simulink model "mult_cmpl"  (R2023a)
settings: Solver=VariableStepAuto  StartTime=0.0  StopTime=5  RelTol=1e-3
settings Model: Creator=usradmin  LastModifiedBy=usradmin

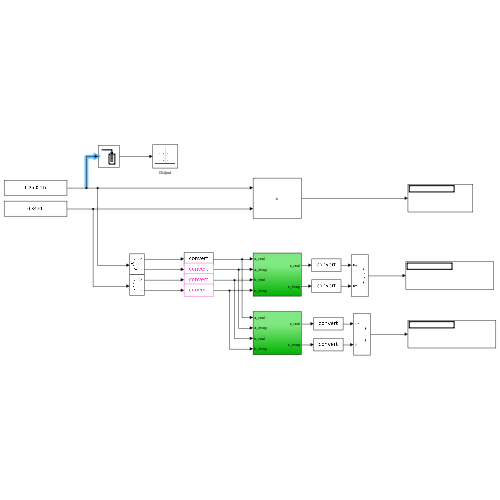
[thumbnail: Simulink's stored preview of the top-level diagram]
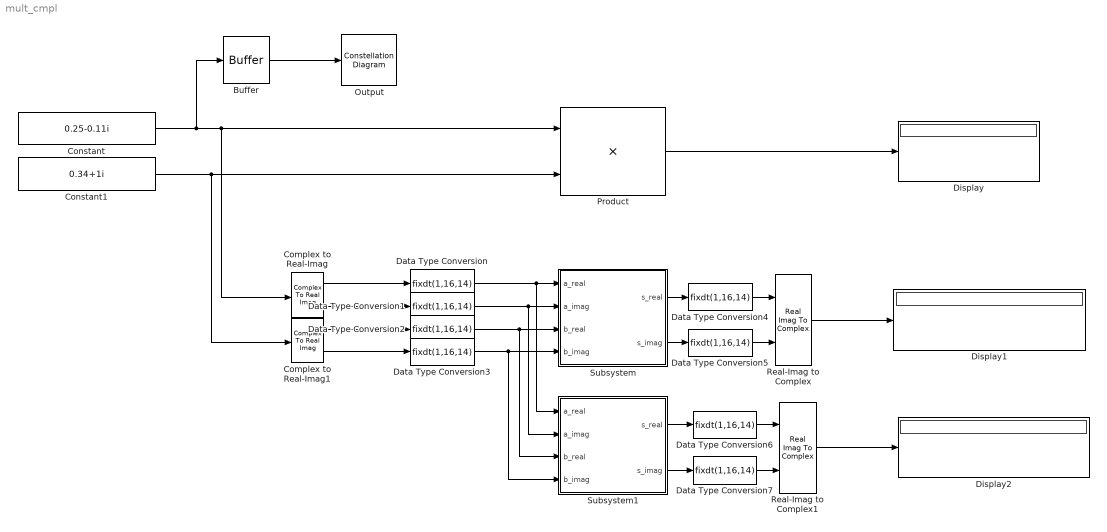
== system mult_cmpl ==
  Buffer : Buffer  N=947*5  OutputFrames=off
  Complex to Real-Imag : ComplexToRealImag
  Complex to Real-Imag1 : ComplexToRealImag
  Constant : Constant  Value=0.25-0.11i
  Constant1 : Constant  Value=0.34+1i
  Data Type Conversion{,1..7} (8 alike) : DataTypeConversion  OutDataTypeStr=fixdt(1,16,14)  SaturateOnIntegerOverflow=off  RndMeth=Floor
  Display : Display
  Display1 : Display
  Display2 : Display
  Output : ConstellationDiagram  WindowPosition=[1891.000000,318.000000,600.000000,600.000000,]  ScopeFrameLocation=window
  Product : Product
  Real-Imag to Complex : RealImagToComplex
  Real-Imag to Complex1 : RealImagToComplex
  Subsystem : Subsystem
  Subsystem1 : Subsystem
  wires:
  Product/1 -> Display/1
  Real-Imag to Complex/1 -> Display1/1
  Constant1/1 -> Complex to Real-Imag1/1, Product/2
  Complex to Real-Imag/1 -> Data Type Conversion/1
  Complex to Real-Imag/2 -> Data Type Conversion1/1
  Complex to Real-Imag1/1 -> Data Type Conversion2/1
  Complex to Real-Imag1/2 -> Data Type Conversion3/1
  Subsystem/1(s_real) -> Data Type Conversion4/1
  Subsystem/2(s_imag) -> Data Type Conversion5/1
  Data Type Conversion/1 -> Subsystem1/1(a_real), Subsystem/1(a_real)
  Data Type Conversion1/1 -> Subsystem1/2(a_imag), Subsystem/2(a_imag)
  Data Type Conversion2/1 -> Subsystem1/3(b_real), Subsystem/3(b_real)
  Data Type Conversion3/1 -> Subsystem1/4(b_imag), Subsystem/4(b_imag)
  Data Type Conversion4/1 -> Real-Imag to Complex/1
  Data Type Conversion5/1 -> Real-Imag to Complex/2
  Data Type Conversion7/1 -> Real-Imag to Complex1/2
  Data Type Conversion6/1 -> Real-Imag to Complex1/1
  Real-Imag to Complex1/1 -> Display2/1
  Subsystem1/1(s_real) -> Data Type Conversion6/1
  Subsystem1/2(s_imag) -> Data Type Conversion7/1
  Buffer/1 -> Output/1
  Constant/1 -> Buffer/1, Complex to Real-Imag/1, Product/1

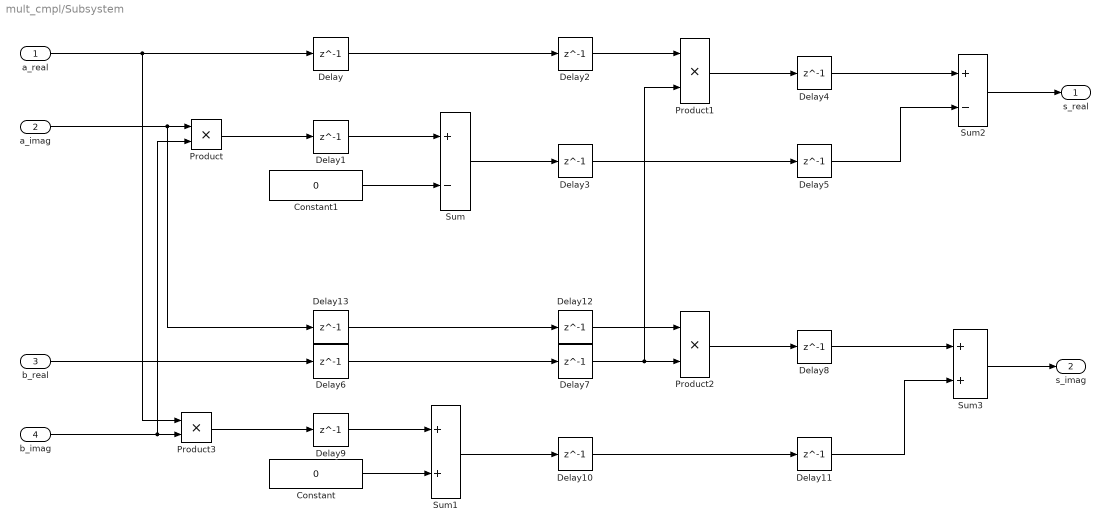
== system mult_cmpl/Subsystem ==
  a_real : Inport
  a_imag : Inport  Port=2
  b_real : Inport  Port=3
  b_imag : Inport  Port=4
  Constant : Constant  Value=0  OutDataTypeStr=fixdt(1,12,11)
  Constant1 : Constant  Value=0  OutDataTypeStr=fixdt(1,12,11)
  Delay{,1..13} (14 alike) : Delay  DelayLength=1  InitialCondition=0
  Product{,1..3} (4 alike) : Product
  Sum : Sum  Inputs=+-
  Sum1 : Sum
  Sum2 : Sum  Inputs=+-
  Sum3 : Sum
  s_real : Outport
  s_imag : Outport  Port=2
  wires:
  a_real/1 -> Delay/1, Product3/1
  a_imag/1 -> Delay13/1, Product/1
  b_imag/1 -> Product3/2, Product/2
  Product/1 -> Delay1/1
  Delay1/1 -> Sum/1
  Delay/1 -> Delay2/1
  Sum/1 -> Delay3/1
  Delay2/1 -> Product1/1
  Product1/1 -> Delay4/1
  Delay4/1 -> Sum2/1
  Delay3/1 -> Delay5/1
  Delay5/1 -> Sum2/2
  Sum2/1 -> s_real/1
  b_real/1 -> Delay6/1
  Delay6/1 -> Delay7/1
  Delay7/1 -> Product1/2, Product2/2
  Product2/1 -> Delay8/1
  Delay8/1 -> Sum3/1
  Sum3/1 -> s_imag/1
  Product3/1 -> Delay9/1
  Delay9/1 -> Sum1/1
  Sum1/1 -> Delay10/1
  Delay10/1 -> Delay11/1
  Delay11/1 -> Sum3/2
  Delay12/1 -> Product2/1
  Delay13/1 -> Delay12/1
  Constant/1 -> Sum1/2
  Constant1/1 -> Sum/2

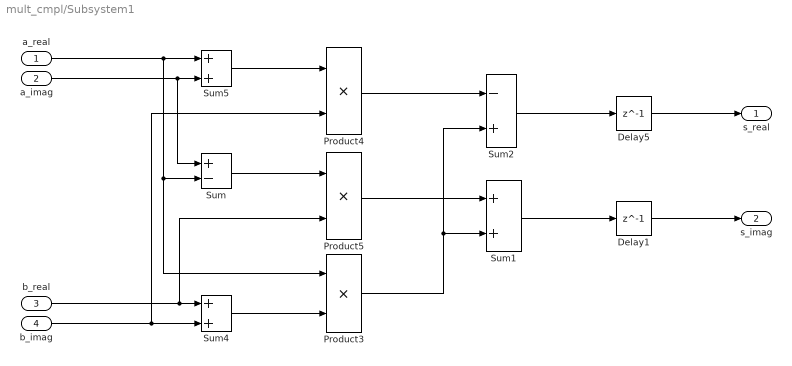
== system mult_cmpl/Subsystem1 ==
  a_real : Inport
  a_imag : Inport  Port=2
  b_real : Inport  Port=3
  b_imag : Inport  Port=4
  Delay1 : Delay  DelayLength=1  InitialCondition=0
  Delay5 : Delay  DelayLength=1  InitialCondition=0
  Product3 : Product
  Product4 : Product
  Product5 : Product
  Sum : Sum  Inputs=+-
  Sum1 : Sum
  Sum2 : Sum  Inputs=-+
  Sum4 : Sum
  Sum5 : Sum
  s_real : Outport
  s_imag : Outport  Port=2
  wires:
  Product3/1 -> Sum1/2, Sum2/2
  Sum1/1 -> Delay1/1
  b_real/1 -> Sum4/1, Product5/2
  Sum2/1 -> Delay5/1
  a_real/1 -> Sum5/1, Product3/1, Sum/2
  b_imag/1 -> Sum4/2, Product4/2
  a_imag/1 -> Sum/1, Sum5/2
  Sum4/1 -> Product3/2
  Sum5/1 -> Product4/1
  Sum/1 -> Product5/1
  Product4/1 -> Sum2/1
  Product5/1 -> Sum1/1
  Delay5/1 -> s_real/1
  Delay1/1 -> s_imag/1
